simulink model "controlsys"  (R2020b)
settings: Solver=VariableStepAuto  StartTime=0.0  StopTime=10.0  RelTol=1e-3
undefined symbols (not defined in the file): a, b, ki, kp, m, ts
settings Model: Creator=mluser  LastModifiedBy=mluser
settings DataIOCC: ExternalInput=[t, stin]  LoadExternalInput=on  SaveFormat=Array  ReturnWorkspaceOutputs=off

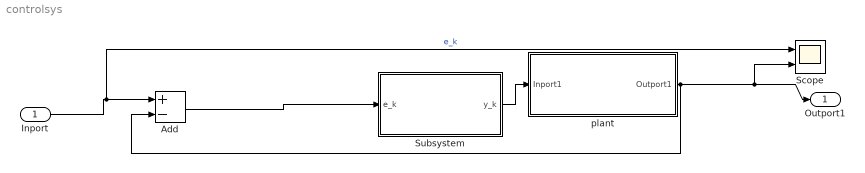
== system controlsys ==
  Inport : Inport
  Add : Sum  Inputs=+-
  Scope : Scope  NumInputPorts=2
  Subsystem : Subsystem
  plant : Subsystem
  Outport1 : Outport
  wires:
  Subsystem/1(y_k) -> plant/1(Inport1)
  plant/1(Outport1) -> Add/2, Scope/2, Outport1/1
  Add/1 -> Subsystem/1(e_k)
  Inport/1 -> Scope/1, Add/1  "e_k"

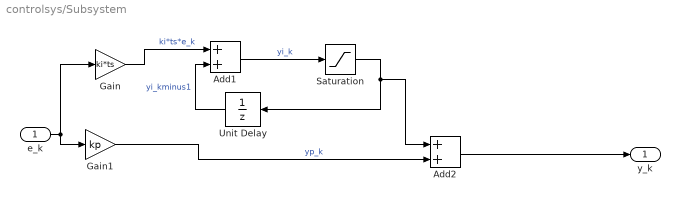
== system controlsys/Subsystem ==
  e_k : Inport
  Add1 : Sum
  Add2 : Sum
  Gain : Gain  Gain=ki*ts
  Gain1 : Gain  Gain=kp
  Saturation : Saturate  UpperLimit=1  LowerLimit=-1
  Unit Delay : UnitDelay  SampleTime=-1  HasFrameUpgradeWarning=on
  y_k : Outport
  wires:
  Saturation/1 -> Add2/1, Unit Delay/1
  Gain/1 -> Add1/1  "ki*ts*e_k"
  Gain1/1 -> Add2/2  "yp_k"
  Unit Delay/1 -> Add1/2  "yi_kminus1"
  e_k/1 -> Gain1/1, Gain/1
  Add1/1 -> Saturation/1  "yi_k"
  Add2/1 -> y_k/1

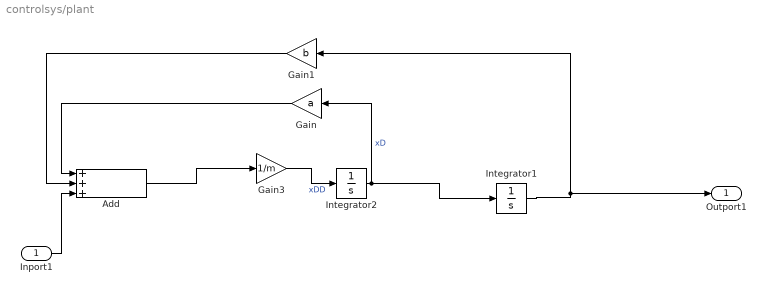
== system controlsys/plant ==
  Inport1 : Inport
  Add : Sum  Inputs=+++
  Gain : Gain  Gain=a
  Gain1 : Gain  Gain=b
  Gain3 : Gain  Gain=1/m
  Integrator1 : Integrator
  Integrator2 : Integrator
  Outport1 : Outport
  wires:
  Gain1/1 -> Add/2
  Gain/1 -> Add/1
  Inport1/1 -> Add/3
  Add/1 -> Gain3/1
  Integrator2/1 -> Gain/1, Integrator1/1  "xD"
  Integrator1/1 -> Outport1/1, Gain1/1
  Gain3/1 -> Integrator2/1  "xDD"
